simulink library "quaternions"  (R2020b)
settings: Solver=VariableStepAuto  StartTime=0.0  StopTime=10.0  RelTol=1e-3
values from neighbouring files (symbols this model uses):
  q0 = eye(4)    [initial_conditions.m]
libraries: vrlib x1, mat_4x4 x1
settings Model: Creator=whitehole  LastModifiedBy=whitehole

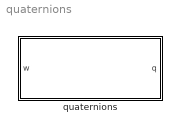
== system quaternions ==
  quaternions : Subsystem

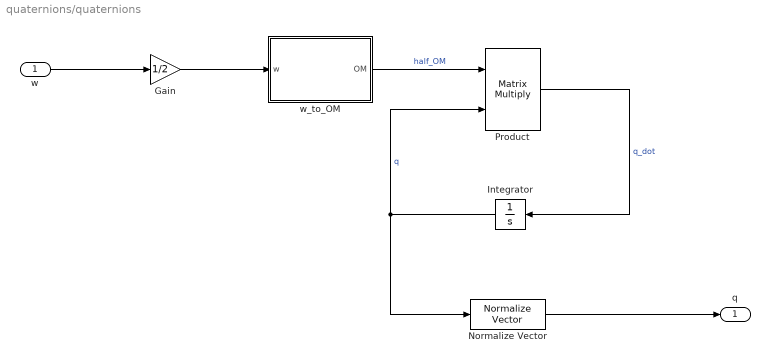
== system quaternions/quaternions ==
  w : Inport
  Gain : Gain  Gain=1/2
  Integrator : Integrator  InitialCondition=q0
  Normalize Vector : vrlib/Utilities/Normalize Vector  maxzero=0
  Product : Product  Multiplication=Matrix(*)
  w_to_OM : Subsystem
  q : Outport
  wires:
  w_to_OM/1(OM) -> Product/1  "half_OM"
  w/1 -> Gain/1
  Product/1 -> Integrator/1  "q_dot"
  Integrator/1 -> Normalize Vector/1, Product/2  "q"
  Gain/1 -> w_to_OM/1(w)
  Normalize Vector/1 -> q/1

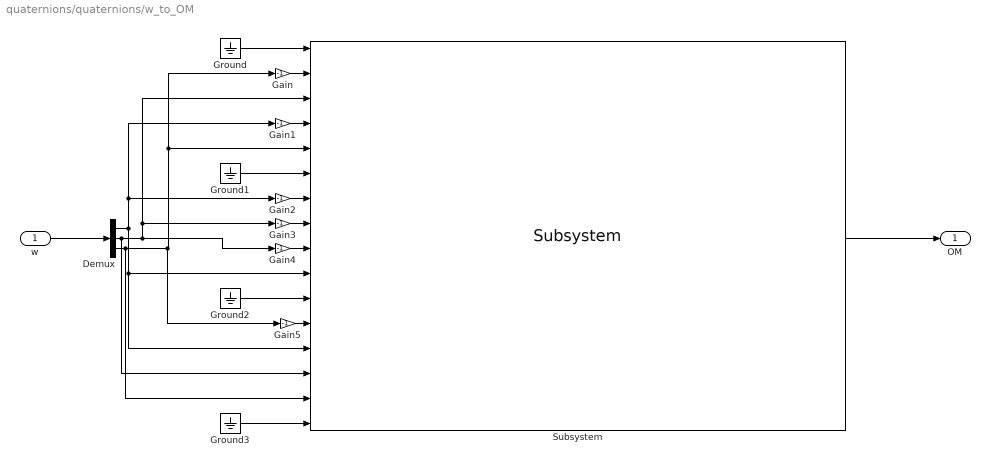
== system quaternions/quaternions/w_to_OM ==
  w : Inport
  Demux : Demux  Outputs=3
  Gain{,1..5} (6 alike) : Gain  Gain=-1
  Ground{,1..3} (4 alike) : Ground
  Subsystem : mat_4x4/Subsystem  SystemSampleTime=-1  VariantActivationTime=update diagram  Latency=0  AutoFrameSizeCalculation=off
  OM : Outport
  wires:
  Subsystem/1 -> OM/1
  w/1 -> Demux/1
  Ground/1 -> Subsystem/1
  Ground1/1 -> Subsystem/6
  Ground2/1 -> Subsystem/11
  Ground3/1 -> Subsystem/16
  Gain/1 -> Subsystem/2
  Demux/3 -> Subsystem/15, Gain5/1, Subsystem/5, Gain/1
  Demux/2 -> Subsystem/14, Gain4/1, Gain3/1, Subsystem/3
  Gain1/1 -> Subsystem/4
  Demux/1 -> Subsystem/13, Subsystem/10, Gain2/1, Gain1/1
  Gain2/1 -> Subsystem/7
  Gain3/1 -> Subsystem/8
  Gain4/1 -> Subsystem/9
  Gain5/1 -> Subsystem/12
